simulink model "MVDR_example_hdl_4x4_systolic"  (R2020a)
settings: Solver=FixedStepDiscrete  StartTime=0.0  StopTime=stoptime  RelTol=1e-3
InitFcn:
  | model_init
values from neighbouring files (symbols this model uses):
  BackSubstitutePrototype = fi(0, matrixdivbacksub_dt)    [model_init.m]
  matrixDivDelay = NumberOfCORDICIterations*10 + 86    [model_init.m]
  movavg_bitshift = nextpow2(sqrt(windowSize))    [model_init.m]
  mvdrPipelineDelay = covMatDelay+movAvgDelay+matrixDivDelay+normResponseDelay    [model_init.m]
  numArrayElements = 4    [model_init.m]
  NumberOfCORDICIterations = matrixdivin_dt.WordLength - 1    [model_init.m]
  srcAngles = [20 60]    [model_init.m]
  sv = step(steeringVector,fc,[scanAngle; 0])    [model_init.m]
  Ts = 1/fs    (= 7.8125e-09)    [model_init.m]
  windowSize = 1024    [model_init.m]
libraries: hdlsllib x249, simulink x44, commfilt2 x4, commrfcorlib x3, commsync2 x3, commrflib2 x2, commrandsrc3 x2, phasedtxrxlib x2, commdigbbndcpm2 x1, dspsolvers x1, embreciprocals x1, commdigbbndpm3 x1
(part 7 of 11)

== system MVDR_example_hdl_4x4_systolic/MVDR HDL/Compute Weight Vector/Matrix Left Divide/CORDIC/4x4 Complex CORDIC Matrix Left Divide/Q'B, R 4x4 Complex CORDIC Systolic Array/Leading Complex Row Rotation/Rotate first element to real/Inverse CORDIC Gain2 ==
  In1 : Inport
  Inverse CORDIC Gain : Gain  Gain=1/prod(sqrt(1+2.^(-2*(0:double(NumberOfCORDICIterations)-1))))  OutDataTypeStr=Inherit: Same as input
  Out1 : Outport  VectorParamsAs1DForOutWhenUnconnected=off
  wires:
  Inverse CORDIC Gain/1 -> Out1/1
  In1/1 -> Inverse CORDIC Gain/1

== system MVDR_example_hdl_4x4_systolic/MVDR HDL/Compute Weight Vector/Matrix Left Divide/CORDIC/4x4 Complex CORDIC Matrix Left Divide/Q'B, R 4x4 Complex CORDIC Systolic Array/Leading Complex Row Rotation/Rotate first element to real/Inverse CORDIC Gain3 ==
  In1 : Inport
  Inverse CORDIC Gain : Gain  Gain=1/prod(sqrt(1+2.^(-2*(0:double(NumberOfCORDICIterations)-1))))  OutDataTypeStr=Inherit: Same as input
  Out1 : Outport  VectorParamsAs1DForOutWhenUnconnected=off
  wires:
  Inverse CORDIC Gain/1 -> Out1/1
  In1/1 -> Inverse CORDIC Gain/1

== system MVDR_example_hdl_4x4_systolic/MVDR HDL/Compute Weight Vector/Matrix Left Divide/CORDIC/4x4 Complex CORDIC Matrix Left Divide/Q'B, R 4x4 Complex CORDIC Systolic Array/Leading Complex Row Rotation/Rotate first element to real/Inverse CORDIC Gain4 ==
  In1 : Inport
  Inverse CORDIC Gain : Gain  Gain=1/prod(sqrt(1+2.^(-2*(0:double(NumberOfCORDICIterations)-1))))  OutDataTypeStr=Inherit: Same as input
  Out1 : Outport  VectorParamsAs1DForOutWhenUnconnected=off
  wires:
  Inverse CORDIC Gain/1 -> Out1/1
  In1/1 -> Inverse CORDIC Gain/1

== system MVDR_example_hdl_4x4_systolic/MVDR HDL/Compute Weight Vector/Matrix Left Divide/CORDIC/4x4 Complex CORDIC Matrix Left Divide/Q'B, R 4x4 Complex CORDIC Systolic Array/Leading Complex Row Rotation/Rotate first element to real/Q'B, R Row Rotations - Real ==
  x : Inport
  y : Inport  Port=2
  u : Inport  Port=3
  v : Inport  Port=4
  validIn : Inport  Port=5
  CORDIC Counter : Subsystem  mask{NumberOfCORDICIterations=NumberOfCORDICIterations}
      mask prompts: NumberOfCORDICIterations "Number of CORDIC Iterations"
  Delay{1..12} (12 alike) : Delay  DelayLength=1
  Delay13 : Delay  DelayLength=1  InitialCondition=true
  MATLAB Function : MATLAB Function  TreatAsAtomicUnit=on
  Same Datatype : Subsystem  TreatAsAtomicUnit=on
  Same Datatype1 : Subsystem  TreatAsAtomicUnit=on
  Same Datatype2 : Subsystem  TreatAsAtomicUnit=on
  Same Datatype3 : Subsystem  TreatAsAtomicUnit=on
  State Control : StateControl  StateControl=Synchronous
  Switch{,1..3} (4 alike) : Switch  Criteria=u2 ~= 0
  x_out : Outport  VectorParamsAs1DForOutWhenUnconnected=off
  y_out : Outport  Port=2  VectorParamsAs1DForOutWhenUnconnected=off
  u_out : Outport  Port=3  VectorParamsAs1DForOutWhenUnconnected=off
  v_out : Outport  Port=4  VectorParamsAs1DForOutWhenUnconnected=off
  validOut : Outport  Port=5  VectorParamsAs1DForOutWhenUnconnected=off
  ready : Outport  Port=6  VectorParamsAs1DForOutWhenUnconnected=off
  wires:
  Delay13/1 -> ready/1
  Delay12/1 -> Delay3/1
  Delay10/1 -> MATLAB Function/5(iteration)
  Delay9/1 -> Switch/2, Switch1/2, Switch2/2, Switch3/2
  Delay8/1 -> Same Datatype2/2(Reference), Switch3/3
  Delay6/1 -> Same Datatype3/2(Reference), Switch2/3
  Delay5/1 -> Same Datatype1/2(Reference), Switch1/3
  Delay4/1 -> Same Datatype/2(Reference), Switch/3
  Delay1/1 -> Same Datatype/1(Data), x_out/1
  Delay2/1 -> Same Datatype1/1(Data), y_out/1
  Delay11/1 -> Same Datatype2/1(Data), v_out/1
  MATLAB Function/1(x_out) -> Delay1/1
  MATLAB Function/2(y_out) -> Delay2/1
  MATLAB Function/3(u_out) -> Delay7/1
  MATLAB Function/4(v_out) -> Delay11/1
  Delay7/1 -> Same Datatype3/1(Data), u_out/1
  Delay3/1 -> validOut/1
  validIn/1 -> CORDIC Counter/1(validIn)
  CORDIC Counter/2(count) -> Delay10/1
  CORDIC Counter/3(last) -> Delay12/1
  CORDIC Counter/4(ready) -> Delay13/1
  Switch/1 -> MATLAB Function/1(x)
  Switch1/1 -> MATLAB Function/2(y)
  Switch2/1 -> MATLAB Function/3(u)
  Switch3/1 -> MATLAB Function/4(v)
  CORDIC Counter/1(count_is_positive) -> Delay9/1
  x/1 -> Delay4/1
  y/1 -> Delay5/1
  u/1 -> Delay6/1
  v/1 -> Delay8/1
  Same Datatype/1(DataOut) -> Switch/1
  Same Datatype1/1(DataOut) -> Switch1/1
  Same Datatype3/1(DataOut) -> Switch2/1
  Same Datatype2/1(DataOut) -> Switch3/1

== system MVDR_example_hdl_4x4_systolic/MVDR HDL/Compute Weight Vector/Matrix Left Divide/CORDIC/4x4 Complex CORDIC Matrix Left Divide/Q'B, R 4x4 Complex CORDIC Systolic Array/Leading Complex Row Rotation/Rotate first element to real/ValidIn to Ready Logic with Delay ==
  readyIn : Inport
  validIn * z^-1 : Inport  Port=2
  validIn : Inport  Port=3
  AND : Logic  IconShape=distinctive  AllPortsSameDT=off  OutDataTypeStr=boolean
  AND1 : Logic  IconShape=distinctive  AllPortsSameDT=off  OutDataTypeStr=boolean
  NOT : Logic  Operator=NOT  IconShape=distinctive  AllPortsSameDT=off  OutDataTypeStr=boolean
  NOT1 : Logic  Operator=NOT  IconShape=distinctive  AllPortsSameDT=off  OutDataTypeStr=boolean
  readyOut : Outport  VectorParamsAs1DForOutWhenUnconnected=off
  wires:
  validIn * z^-1/1 -> NOT/1
  validIn/1 -> NOT1/1
  readyIn/1 -> AND/1
  AND1/1 -> readyOut/1
  NOT1/1 -> AND1/2
  NOT/1 -> AND/2
  AND/1 -> AND1/1

== system MVDR_example_hdl_4x4_systolic/MVDR HDL/Compute Weight Vector/Matrix Left Divide/CORDIC/4x4 Complex CORDIC Matrix Left Divide/Q'B, R 4x4 Complex CORDIC Systolic Array/Leading Complex Row Rotation/Rotate first element to real - 1/Inverse CORDIC Gain1 ==
  In1 : Inport
  Inverse CORDIC Gain : Gain  Gain=1/prod(sqrt(1+2.^(-2*(0:double(NumberOfCORDICIterations)-1))))  OutDataTypeStr=Inherit: Same as input
  Out1 : Outport  VectorParamsAs1DForOutWhenUnconnected=off
  wires:
  Inverse CORDIC Gain/1 -> Out1/1
  In1/1 -> Inverse CORDIC Gain/1

== system MVDR_example_hdl_4x4_systolic/MVDR HDL/Compute Weight Vector/Matrix Left Divide/CORDIC/4x4 Complex CORDIC Matrix Left Divide/Q'B, R 4x4 Complex CORDIC Systolic Array/Leading Complex Row Rotation/Rotate first element to real - 1/Inverse CORDIC Gain2 ==
  In1 : Inport
  Inverse CORDIC Gain : Gain  Gain=1/prod(sqrt(1+2.^(-2*(0:double(NumberOfCORDICIterations)-1))))  OutDataTypeStr=Inherit: Same as input
  Out1 : Outport  VectorParamsAs1DForOutWhenUnconnected=off
  wires:
  Inverse CORDIC Gain/1 -> Out1/1
  In1/1 -> Inverse CORDIC Gain/1

== system MVDR_example_hdl_4x4_systolic/MVDR HDL/Compute Weight Vector/Matrix Left Divide/CORDIC/4x4 Complex CORDIC Matrix Left Divide/Q'B, R 4x4 Complex CORDIC Systolic Array/Leading Complex Row Rotation/Rotate first element to real - 1/Inverse CORDIC Gain3 ==
  In1 : Inport
  Inverse CORDIC Gain : Gain  Gain=1/prod(sqrt(1+2.^(-2*(0:double(NumberOfCORDICIterations)-1))))  OutDataTypeStr=Inherit: Same as input
  Out1 : Outport  VectorParamsAs1DForOutWhenUnconnected=off
  wires:
  Inverse CORDIC Gain/1 -> Out1/1
  In1/1 -> Inverse CORDIC Gain/1

== system MVDR_example_hdl_4x4_systolic/MVDR HDL/Compute Weight Vector/Matrix Left Divide/CORDIC/4x4 Complex CORDIC Matrix Left Divide/Q'B, R 4x4 Complex CORDIC Systolic Array/Leading Complex Row Rotation/Rotate first element to real - 1/Inverse CORDIC Gain4 ==
  In1 : Inport
  Inverse CORDIC Gain : Gain  Gain=1/prod(sqrt(1+2.^(-2*(0:double(NumberOfCORDICIterations)-1))))  OutDataTypeStr=Inherit: Same as input
  Out1 : Outport  VectorParamsAs1DForOutWhenUnconnected=off
  wires:
  Inverse CORDIC Gain/1 -> Out1/1
  In1/1 -> Inverse CORDIC Gain/1

== system MVDR_example_hdl_4x4_systolic/MVDR HDL/Compute Weight Vector/Matrix Left Divide/CORDIC/4x4 Complex CORDIC Matrix Left Divide/Q'B, R 4x4 Complex CORDIC Systolic Array/Leading Complex Row Rotation/Rotate first element to real - 1/Q'B, R Row Rotations - Real ==
  x : Inport
  y : Inport  Port=2
  u : Inport  Port=3
  v : Inport  Port=4
  validIn : Inport  Port=5
  CORDIC Counter : Subsystem  mask{NumberOfCORDICIterations=NumberOfCORDICIterations}
      mask prompts: NumberOfCORDICIterations "Number of CORDIC Iterations"
  Delay{1..12} (12 alike) : Delay  DelayLength=1
  Delay13 : Delay  DelayLength=1  InitialCondition=true
  MATLAB Function : MATLAB Function  TreatAsAtomicUnit=on
  Same Datatype : Subsystem  TreatAsAtomicUnit=on
  Same Datatype1 : Subsystem  TreatAsAtomicUnit=on
  Same Datatype2 : Subsystem  TreatAsAtomicUnit=on
  Same Datatype3 : Subsystem  TreatAsAtomicUnit=on
  State Control : StateControl  StateControl=Synchronous
  Switch{,1..3} (4 alike) : Switch  Criteria=u2 ~= 0
  x_out : Outport  VectorParamsAs1DForOutWhenUnconnected=off
  y_out : Outport  Port=2  VectorParamsAs1DForOutWhenUnconnected=off
  u_out : Outport  Port=3  VectorParamsAs1DForOutWhenUnconnected=off
  v_out : Outport  Port=4  VectorParamsAs1DForOutWhenUnconnected=off
  validOut : Outport  Port=5  VectorParamsAs1DForOutWhenUnconnected=off
  ready : Outport  Port=6  VectorParamsAs1DForOutWhenUnconnected=off
  wires:
  Delay13/1 -> ready/1
  Delay12/1 -> Delay3/1
  Delay10/1 -> MATLAB Function/5(iteration)
  Delay9/1 -> Switch/2, Switch1/2, Switch2/2, Switch3/2
  Delay8/1 -> Same Datatype2/2(Reference), Switch3/3
  Delay6/1 -> Same Datatype3/2(Reference), Switch2/3
  Delay5/1 -> Same Datatype1/2(Reference), Switch1/3
  Delay4/1 -> Same Datatype/2(Reference), Switch/3
  Delay1/1 -> Same Datatype/1(Data), x_out/1
  Delay2/1 -> Same Datatype1/1(Data), y_out/1
  Delay11/1 -> Same Datatype2/1(Data), v_out/1
  MATLAB Function/1(x_out) -> Delay1/1
  MATLAB Function/2(y_out) -> Delay2/1
  MATLAB Function/3(u_out) -> Delay7/1
  MATLAB Function/4(v_out) -> Delay11/1
  Delay7/1 -> Same Datatype3/1(Data), u_out/1
  Delay3/1 -> validOut/1
  validIn/1 -> CORDIC Counter/1(validIn)
  CORDIC Counter/2(count) -> Delay10/1
  CORDIC Counter/3(last) -> Delay12/1
  CORDIC Counter/4(ready) -> Delay13/1
  Switch/1 -> MATLAB Function/1(x)
  Switch1/1 -> MATLAB Function/2(y)
  Switch2/1 -> MATLAB Function/3(u)
  Switch3/1 -> MATLAB Function/4(v)
  CORDIC Counter/1(count_is_positive) -> Delay9/1
  x/1 -> Delay4/1
  y/1 -> Delay5/1
  u/1 -> Delay6/1
  v/1 -> Delay8/1
  Same Datatype/1(DataOut) -> Switch/1
  Same Datatype1/1(DataOut) -> Switch1/1
  Same Datatype3/1(DataOut) -> Switch2/1
  Same Datatype2/1(DataOut) -> Switch3/1

== system MVDR_example_hdl_4x4_systolic/MVDR HDL/Compute Weight Vector/Matrix Left Divide/CORDIC/4x4 Complex CORDIC Matrix Left Divide/Q'B, R 4x4 Complex CORDIC Systolic Array/Leading Complex Row Rotation/Rotate first element to real - 1/ValidIn to Ready Logic with Delay ==
  readyIn : Inport
  validIn * z^-1 : Inport  Port=2
  validIn : Inport  Port=3
  AND : Logic  IconShape=distinctive  AllPortsSameDT=off  OutDataTypeStr=boolean
  AND1 : Logic  IconShape=distinctive  AllPortsSameDT=off  OutDataTypeStr=boolean
  NOT : Logic  Operator=NOT  IconShape=distinctive  AllPortsSameDT=off  OutDataTypeStr=boolean
  NOT1 : Logic  Operator=NOT  IconShape=distinctive  AllPortsSameDT=off  OutDataTypeStr=boolean
  readyOut : Outport  VectorParamsAs1DForOutWhenUnconnected=off
  wires:
  validIn * z^-1/1 -> NOT/1
  validIn/1 -> NOT1/1
  readyIn/1 -> AND/1
  AND1/1 -> readyOut/1
  NOT1/1 -> AND1/2
  NOT/1 -> AND/2
  AND/1 -> AND1/1

== system MVDR_example_hdl_4x4_systolic/MVDR HDL/Compute Weight Vector/Matrix Left Divide/CORDIC/4x4 Complex CORDIC Matrix Left Divide/Q'B, R 4x4 Complex CORDIC Systolic Array/Leading Complex Row Rotation - 2/Q'B, R Row Rotations - Complex/CORDIC Counter ==
  validIn : Inport
  Compare To Constant : simulink/Logic and Bit Operations/Compare To Constant  relop===  const=NumberOfCORDICIterations-1  OutDataTypeStr=boolean
  Compare To Zero : simulink/Logic and Bit Operations/Compare To Zero  relop=>  OutDataTypeStr=boolean
  HDL Counter1 : hdlsllib/Sources/HDL Counter  CountType=Count limited  CountInit=0  CountStep=1  CountMax=NumberOfCORDICIterations-1  CountFromType=Initial value  CountFrom=0  CountResetPort=off  CountLoadPort=off  CountEnbPort=on  CountDirPort=off  CountDataType=Unsigned  CountWordLen=nextpow2(NumberOfCORDICIterations)  CountFracLen=0  CountSampTime=1
  OR : Logic  Operator=OR  IconShape=distinctive  AllPortsSameDT=off  OutDataTypeStr=boolean
  SR_latch : Subsystem
  State Control : StateControl  StateControl=Synchronous
  ValidIn to Ready Logic : Subsystem
  count_is_positive : Outport  VectorParamsAs1DForOutWhenUnconnected=off
  count : Outport  Port=2  VectorParamsAs1DForOutWhenUnconnected=off
  last : Outport  Port=3  VectorParamsAs1DForOutWhenUnconnected=off
  ready : Outport  Port=4  VectorParamsAs1DForOutWhenUnconnected=off
  wires:
  HDL Counter1/1 -> Compare To Zero/1, count/1, Compare To Constant/1  "count"
  OR/1 -> HDL Counter1/1
  Compare To Zero/1 -> count_is_positive/1, OR/1
  Compare To Constant/1 -> SR_latch/1(S), last/1
  validIn/1 -> ValidIn to Ready Logic/2(validIn), SR_latch/2(R), OR/2
  SR_latch/1(Q) -> ValidIn to Ready Logic/1(readyIn)  "ready"
  ValidIn to Ready Logic/1(readyOut) -> ready/1

== system MVDR_example_hdl_4x4_systolic/MVDR HDL/Compute Weight Vector/Matrix Left Divide/CORDIC/4x4 Complex CORDIC Matrix Left Divide/Q'B, R 4x4 Complex CORDIC Systolic Array/Leading Complex Row Rotation - 2/Q'B, R Row Rotations - Complex/Same Datatype ==
  Data : Inport
  Reference : Inport  Port=2
  Data Type Duplicate : DataTypeDuplicate
  DataOut : Outport  VectorParamsAs1DForOutWhenUnconnected=off
  wires:
  Data/1 -> Data Type Duplicate/1, DataOut/1
  Reference/1 -> Data Type Duplicate/2

== system MVDR_example_hdl_4x4_systolic/MVDR HDL/Compute Weight Vector/Matrix Left Divide/CORDIC/4x4 Complex CORDIC Matrix Left Divide/Q'B, R 4x4 Complex CORDIC Systolic Array/Leading Complex Row Rotation - 2/Q'B, R Row Rotations - Complex/Same Datatype1 ==
  Data : Inport
  Reference : Inport  Port=2
  Data Type Duplicate : DataTypeDuplicate
  DataOut : Outport  VectorParamsAs1DForOutWhenUnconnected=off
  wires:
  Data/1 -> Data Type Duplicate/1, DataOut/1
  Reference/1 -> Data Type Duplicate/2

== system MVDR_example_hdl_4x4_systolic/MVDR HDL/Compute Weight Vector/Matrix Left Divide/CORDIC/4x4 Complex CORDIC Matrix Left Divide/Q'B, R 4x4 Complex CORDIC Systolic Array/Leading Complex Row Rotation - 2/Q'B, R Row Rotations - Complex/Same Datatype2 ==
  Data : Inport
  Reference : Inport  Port=2
  Data Type Duplicate : DataTypeDuplicate
  DataOut : Outport  VectorParamsAs1DForOutWhenUnconnected=off
  wires:
  Data/1 -> Data Type Duplicate/1, DataOut/1
  Reference/1 -> Data Type Duplicate/2

== system MVDR_example_hdl_4x4_systolic/MVDR HDL/Compute Weight Vector/Matrix Left Divide/CORDIC/4x4 Complex CORDIC Matrix Left Divide/Q'B, R 4x4 Complex CORDIC Systolic Array/Leading Complex Row Rotation - 2/Q'B, R Row Rotations - Complex/Same Datatype3 ==
  Data : Inport
  Reference : Inport  Port=2
  Data Type Duplicate : DataTypeDuplicate
  DataOut : Outport  VectorParamsAs1DForOutWhenUnconnected=off
  wires:
  Data/1 -> Data Type Duplicate/1, DataOut/1
  Reference/1 -> Data Type Duplicate/2

== system MVDR_example_hdl_4x4_systolic/MVDR HDL/Compute Weight Vector/Matrix Left Divide/CORDIC/4x4 Complex CORDIC Matrix Left Divide/Q'B, R 4x4 Complex CORDIC Systolic Array/Leading Complex Row Rotation - 2/Rotate first element to real/Inverse CORDIC Gain1 ==
  In1 : Inport
  Inverse CORDIC Gain : Gain  Gain=1/prod(sqrt(1+2.^(-2*(0:double(NumberOfCORDICIterations)-1))))  OutDataTypeStr=Inherit: Same as input
  Out1 : Outport  VectorParamsAs1DForOutWhenUnconnected=off
  wires:
  Inverse CORDIC Gain/1 -> Out1/1
  In1/1 -> Inverse CORDIC Gain/1

== system MVDR_example_hdl_4x4_systolic/MVDR HDL/Compute Weight Vector/Matrix Left Divide/CORDIC/4x4 Complex CORDIC Matrix Left Divide/Q'B, R 4x4 Complex CORDIC Systolic Array/Leading Complex Row Rotation - 2/Rotate first element to real/Inverse CORDIC Gain2 ==
  In1 : Inport
  Inverse CORDIC Gain : Gain  Gain=1/prod(sqrt(1+2.^(-2*(0:double(NumberOfCORDICIterations)-1))))  OutDataTypeStr=Inherit: Same as input
  Out1 : Outport  VectorParamsAs1DForOutWhenUnconnected=off
  wires:
  Inverse CORDIC Gain/1 -> Out1/1
  In1/1 -> Inverse CORDIC Gain/1

== system MVDR_example_hdl_4x4_systolic/MVDR HDL/Compute Weight Vector/Matrix Left Divide/CORDIC/4x4 Complex CORDIC Matrix Left Divide/Q'B, R 4x4 Complex CORDIC Systolic Array/Leading Complex Row Rotation - 2/Rotate first element to real/Inverse CORDIC Gain3 ==
  In1 : Inport
  Inverse CORDIC Gain : Gain  Gain=1/prod(sqrt(1+2.^(-2*(0:double(NumberOfCORDICIterations)-1))))  OutDataTypeStr=Inherit: Same as input
  Out1 : Outport  VectorParamsAs1DForOutWhenUnconnected=off
  wires:
  Inverse CORDIC Gain/1 -> Out1/1
  In1/1 -> Inverse CORDIC Gain/1

== system MVDR_example_hdl_4x4_systolic/MVDR HDL/Compute Weight Vector/Matrix Left Divide/CORDIC/4x4 Complex CORDIC Matrix Left Divide/Q'B, R 4x4 Complex CORDIC Systolic Array/Leading Complex Row Rotation - 2/Rotate first element to real/Inverse CORDIC Gain4 ==
  In1 : Inport
  Inverse CORDIC Gain : Gain  Gain=1/prod(sqrt(1+2.^(-2*(0:double(NumberOfCORDICIterations)-1))))  OutDataTypeStr=Inherit: Same as input
  Out1 : Outport  VectorParamsAs1DForOutWhenUnconnected=off
  wires:
  Inverse CORDIC Gain/1 -> Out1/1
  In1/1 -> Inverse CORDIC Gain/1

== system MVDR_example_hdl_4x4_systolic/MVDR HDL/Compute Weight Vector/Matrix Left Divide/CORDIC/4x4 Complex CORDIC Matrix Left Divide/Q'B, R 4x4 Complex CORDIC Systolic Array/Leading Complex Row Rotation - 2/Rotate first element to real/Q'B, R Row Rotations - Real ==
  x : Inport
  y : Inport  Port=2
  u : Inport  Port=3
  v : Inport  Port=4
  validIn : Inport  Port=5
  CORDIC Counter : Subsystem  mask{NumberOfCORDICIterations=NumberOfCORDICIterations}
      mask prompts: NumberOfCORDICIterations "Number of CORDIC Iterations"
  Delay{1..12} (12 alike) : Delay  DelayLength=1
  Delay13 : Delay  DelayLength=1  InitialCondition=true
  MATLAB Function : MATLAB Function  TreatAsAtomicUnit=on
  Same Datatype : Subsystem  TreatAsAtomicUnit=on
  Same Datatype1 : Subsystem  TreatAsAtomicUnit=on
  Same Datatype2 : Subsystem  TreatAsAtomicUnit=on
  Same Datatype3 : Subsystem  TreatAsAtomicUnit=on
  State Control : StateControl  StateControl=Synchronous
  Switch{,1..3} (4 alike) : Switch  Criteria=u2 ~= 0
  x_out : Outport  VectorParamsAs1DForOutWhenUnconnected=off
  y_out : Outport  Port=2  VectorParamsAs1DForOutWhenUnconnected=off
  u_out : Outport  Port=3  VectorParamsAs1DForOutWhenUnconnected=off
  v_out : Outport  Port=4  VectorParamsAs1DForOutWhenUnconnected=off
  validOut : Outport  Port=5  VectorParamsAs1DForOutWhenUnconnected=off
  ready : Outport  Port=6  VectorParamsAs1DForOutWhenUnconnected=off
  wires:
  Delay13/1 -> ready/1
  Delay12/1 -> Delay3/1
  Delay10/1 -> MATLAB Function/5(iteration)
  Delay9/1 -> Switch/2, Switch1/2, Switch2/2, Switch3/2
  Delay8/1 -> Same Datatype2/2(Reference), Switch3/3
  Delay6/1 -> Same Datatype3/2(Reference), Switch2/3
  Delay5/1 -> Same Datatype1/2(Reference), Switch1/3
  Delay4/1 -> Same Datatype/2(Reference), Switch/3
  Delay1/1 -> Same Datatype/1(Data), x_out/1
  Delay2/1 -> Same Datatype1/1(Data), y_out/1
  Delay11/1 -> Same Datatype2/1(Data), v_out/1
  MATLAB Function/1(x_out) -> Delay1/1
  MATLAB Function/2(y_out) -> Delay2/1
  MATLAB Function/3(u_out) -> Delay7/1
  MATLAB Function/4(v_out) -> Delay11/1
  Delay7/1 -> Same Datatype3/1(Data), u_out/1
  Delay3/1 -> validOut/1
  validIn/1 -> CORDIC Counter/1(validIn)
  CORDIC Counter/2(count) -> Delay10/1
  CORDIC Counter/3(last) -> Delay12/1
  CORDIC Counter/4(ready) -> Delay13/1
  Switch/1 -> MATLAB Function/1(x)
  Switch1/1 -> MATLAB Function/2(y)
  Switch2/1 -> MATLAB Function/3(u)
  Switch3/1 -> MATLAB Function/4(v)
  CORDIC Counter/1(count_is_positive) -> Delay9/1
  x/1 -> Delay4/1
  y/1 -> Delay5/1
  u/1 -> Delay6/1
  v/1 -> Delay8/1
  Same Datatype/1(DataOut) -> Switch/1
  Same Datatype1/1(DataOut) -> Switch1/1
  Same Datatype3/1(DataOut) -> Switch2/1
  Same Datatype2/1(DataOut) -> Switch3/1

== system MVDR_example_hdl_4x4_systolic/MVDR HDL/Compute Weight Vector/Matrix Left Divide/CORDIC/4x4 Complex CORDIC Matrix Left Divide/Q'B, R 4x4 Complex CORDIC Systolic Array/Leading Complex Row Rotation - 2/Rotate first element to real/ValidIn to Ready Logic with Delay ==
  readyIn : Inport
  validIn * z^-1 : Inport  Port=2
  validIn : Inport  Port=3
  AND : Logic  IconShape=distinctive  AllPortsSameDT=off  OutDataTypeStr=boolean
  AND1 : Logic  IconShape=distinctive  AllPortsSameDT=off  OutDataTypeStr=boolean
  NOT : Logic  Operator=NOT  IconShape=distinctive  AllPortsSameDT=off  OutDataTypeStr=boolean
  NOT1 : Logic  Operator=NOT  IconShape=distinctive  AllPortsSameDT=off  OutDataTypeStr=boolean
  readyOut : Outport  VectorParamsAs1DForOutWhenUnconnected=off
  wires:
  validIn * z^-1/1 -> NOT/1
  validIn/1 -> NOT1/1
  readyIn/1 -> AND/1
  AND1/1 -> readyOut/1
  NOT1/1 -> AND1/2
  NOT/1 -> AND/2
  AND/1 -> AND1/1

== system MVDR_example_hdl_4x4_systolic/MVDR HDL/Compute Weight Vector/Matrix Left Divide/CORDIC/4x4 Complex CORDIC Matrix Left Divide/Q'B, R 4x4 Complex CORDIC Systolic Array/Leading Complex Row Rotation - 2/Rotate first element to real - 1/Inverse CORDIC Gain1 ==
  In1 : Inport
  Inverse CORDIC Gain : Gain  Gain=1/prod(sqrt(1+2.^(-2*(0:double(NumberOfCORDICIterations)-1))))  OutDataTypeStr=Inherit: Same as input
  Out1 : Outport  VectorParamsAs1DForOutWhenUnconnected=off
  wires:
  Inverse CORDIC Gain/1 -> Out1/1
  In1/1 -> Inverse CORDIC Gain/1

== system MVDR_example_hdl_4x4_systolic/MVDR HDL/Compute Weight Vector/Matrix Left Divide/CORDIC/4x4 Complex CORDIC Matrix Left Divide/Q'B, R 4x4 Complex CORDIC Systolic Array/Leading Complex Row Rotation - 2/Rotate first element to real - 1/Inverse CORDIC Gain2 ==
  In1 : Inport
  Inverse CORDIC Gain : Gain  Gain=1/prod(sqrt(1+2.^(-2*(0:double(NumberOfCORDICIterations)-1))))  OutDataTypeStr=Inherit: Same as input
  Out1 : Outport  VectorParamsAs1DForOutWhenUnconnected=off
  wires:
  Inverse CORDIC Gain/1 -> Out1/1
  In1/1 -> Inverse CORDIC Gain/1

== system MVDR_example_hdl_4x4_systolic/MVDR HDL/Compute Weight Vector/Matrix Left Divide/CORDIC/4x4 Complex CORDIC Matrix Left Divide/Q'B, R 4x4 Complex CORDIC Systolic Array/Leading Complex Row Rotation - 2/Rotate first element to real - 1/Inverse CORDIC Gain3 ==
  In1 : Inport
  Inverse CORDIC Gain : Gain  Gain=1/prod(sqrt(1+2.^(-2*(0:double(NumberOfCORDICIterations)-1))))  OutDataTypeStr=Inherit: Same as input
  Out1 : Outport  VectorParamsAs1DForOutWhenUnconnected=off
  wires:
  Inverse CORDIC Gain/1 -> Out1/1
  In1/1 -> Inverse CORDIC Gain/1

== system MVDR_example_hdl_4x4_systolic/MVDR HDL/Compute Weight Vector/Matrix Left Divide/CORDIC/4x4 Complex CORDIC Matrix Left Divide/Q'B, R 4x4 Complex CORDIC Systolic Array/Leading Complex Row Rotation - 2/Rotate first element to real - 1/Inverse CORDIC Gain4 ==
  In1 : Inport
  Inverse CORDIC Gain : Gain  Gain=1/prod(sqrt(1+2.^(-2*(0:double(NumberOfCORDICIterations)-1))))  OutDataTypeStr=Inherit: Same as input
  Out1 : Outport  VectorParamsAs1DForOutWhenUnconnected=off
  wires:
  Inverse CORDIC Gain/1 -> Out1/1
  In1/1 -> Inverse CORDIC Gain/1

== system MVDR_example_hdl_4x4_systolic/MVDR HDL/Compute Weight Vector/Matrix Left Divide/CORDIC/4x4 Complex CORDIC Matrix Left Divide/Q'B, R 4x4 Complex CORDIC Systolic Array/Leading Complex Row Rotation - 2/Rotate first element to real - 1/Q'B, R Row Rotations - Real ==
  x : Inport
  y : Inport  Port=2
  u : Inport  Port=3
  v : Inport  Port=4
  validIn : Inport  Port=5
  CORDIC Counter : Subsystem  mask{NumberOfCORDICIterations=NumberOfCORDICIterations}
      mask prompts: NumberOfCORDICIterations "Number of CORDIC Iterations"
  Delay{1..12} (12 alike) : Delay  DelayLength=1
  Delay13 : Delay  DelayLength=1  InitialCondition=true
  MATLAB Function : MATLAB Function  TreatAsAtomicUnit=on
  Same Datatype : Subsystem  TreatAsAtomicUnit=on
  Same Datatype1 : Subsystem  TreatAsAtomicUnit=on
  Same Datatype2 : Subsystem  TreatAsAtomicUnit=on
  Same Datatype3 : Subsystem  TreatAsAtomicUnit=on
  State Control : StateControl  StateControl=Synchronous
  Switch{,1..3} (4 alike) : Switch  Criteria=u2 ~= 0
  x_out : Outport  VectorParamsAs1DForOutWhenUnconnected=off
  y_out : Outport  Port=2  VectorParamsAs1DForOutWhenUnconnected=off
  u_out : Outport  Port=3  VectorParamsAs1DForOutWhenUnconnected=off
  v_out : Outport  Port=4  VectorParamsAs1DForOutWhenUnconnected=off
  validOut : Outport  Port=5  VectorParamsAs1DForOutWhenUnconnected=off
  ready : Outport  Port=6  VectorParamsAs1DForOutWhenUnconnected=off
  wires:
  Same Datatype2/1(DataOut) -> Switch3/1
  Same Datatype3/1(DataOut) -> Switch2/1
  Same Datatype1/1(DataOut) -> Switch1/1
  Same Datatype/1(DataOut) -> Switch/1
  v/1 -> Delay8/1
  u/1 -> Delay6/1
  y/1 -> Delay5/1
  x/1 -> Delay4/1
  CORDIC Counter/1(count_is_positive) -> Delay9/1
  Switch3/1 -> MATLAB Function/4(v)
  Switch2/1 -> MATLAB Function/3(u)
  Switch1/1 -> MATLAB Function/2(y)
  Switch/1 -> MATLAB Function/1(x)
  CORDIC Counter/4(ready) -> Delay13/1
  CORDIC Counter/3(last) -> Delay12/1
  CORDIC Counter/2(count) -> Delay10/1
  validIn/1 -> CORDIC Counter/1(validIn)
  Delay3/1 -> validOut/1
  Delay7/1 -> u_out/1, Same Datatype3/1(Data)
  MATLAB Function/4(v_out) -> Delay11/1
  MATLAB Function/3(u_out) -> Delay7/1
  MATLAB Function/2(y_out) -> Delay2/1
  MATLAB Function/1(x_out) -> Delay1/1
  Delay11/1 -> v_out/1, Same Datatype2/1(Data)
  Delay2/1 -> y_out/1, Same Datatype1/1(Data)
  Delay1/1 -> x_out/1, Same Datatype/1(Data)
  Delay4/1 -> Switch/3, Same Datatype/2(Reference)
  Delay5/1 -> Switch1/3, Same Datatype1/2(Reference)
  Delay6/1 -> Switch2/3, Same Datatype3/2(Reference)
  Delay8/1 -> Switch3/3, Same Datatype2/2(Reference)
  Delay9/1 -> Switch3/2, Switch2/2, Switch1/2, Switch/2
  Delay10/1 -> MATLAB Function/5(iteration)
  Delay12/1 -> Delay3/1
  Delay13/1 -> ready/1

== system MVDR_example_hdl_4x4_systolic/MVDR HDL/Compute Weight Vector/Matrix Left Divide/CORDIC/4x4 Complex CORDIC Matrix Left Divide/Q'B, R 4x4 Complex CORDIC Systolic Array/Leading Complex Row Rotation - 2/Rotate first element to real - 1/ValidIn to Ready Logic with Delay ==
  readyIn : Inport
  validIn * z^-1 : Inport  Port=2
  validIn : Inport  Port=3
  AND : Logic  IconShape=distinctive  AllPortsSameDT=off  OutDataTypeStr=boolean
  AND1 : Logic  IconShape=distinctive  AllPortsSameDT=off  OutDataTypeStr=boolean
  NOT : Logic  Operator=NOT  IconShape=distinctive  AllPortsSameDT=off  OutDataTypeStr=boolean
  NOT1 : Logic  Operator=NOT  IconShape=distinctive  AllPortsSameDT=off  OutDataTypeStr=boolean
  readyOut : Outport  VectorParamsAs1DForOutWhenUnconnected=off
  wires:
  validIn * z^-1/1 -> NOT/1
  validIn/1 -> NOT1/1
  readyIn/1 -> AND/1
  AND1/1 -> readyOut/1
  NOT1/1 -> AND1/2
  NOT/1 -> AND/2
  AND/1 -> AND1/1

== system MVDR_example_hdl_4x4_systolic/MVDR HDL/Compute Weight Vector/Matrix Left Divide/CORDIC/4x4 Complex CORDIC Matrix Left Divide/Q'B, R 4x4 Complex CORDIC Systolic Array/Leading Complex Row Rotation - 3/Q'B, R Row Rotations - Complex/CORDIC Counter ==
  validIn : Inport
  Compare To Constant : simulink/Logic and Bit Operations/Compare To Constant  relop===  const=NumberOfCORDICIterations-1  OutDataTypeStr=boolean
  Compare To Zero : simulink/Logic and Bit Operations/Compare To Zero  relop=>  OutDataTypeStr=boolean
  HDL Counter1 : hdlsllib/Sources/HDL Counter  CountType=Count limited  CountInit=0  CountStep=1  CountMax=NumberOfCORDICIterations-1  CountFromType=Initial value  CountFrom=0  CountResetPort=off  CountLoadPort=off  CountEnbPort=on  CountDirPort=off  CountDataType=Unsigned  CountWordLen=nextpow2(NumberOfCORDICIterations)  CountFracLen=0  CountSampTime=1
  OR : Logic  Operator=OR  IconShape=distinctive  AllPortsSameDT=off  OutDataTypeStr=boolean
  SR_latch : Subsystem
  State Control : StateControl  StateControl=Synchronous
  ValidIn to Ready Logic : Subsystem
  count_is_positive : Outport  VectorParamsAs1DForOutWhenUnconnected=off
  count : Outport  Port=2  VectorParamsAs1DForOutWhenUnconnected=off
  last : Outport  Port=3  VectorParamsAs1DForOutWhenUnconnected=off
  ready : Outport  Port=4  VectorParamsAs1DForOutWhenUnconnected=off
  wires:
  ValidIn to Ready Logic/1(readyOut) -> ready/1
  SR_latch/1(Q) -> ValidIn to Ready Logic/1(readyIn)  "ready"
  validIn/1 -> OR/2, SR_latch/2(R), ValidIn to Ready Logic/2(validIn)
  Compare To Constant/1 -> last/1, SR_latch/1(S)
  Compare To Zero/1 -> OR/1, count_is_positive/1
  OR/1 -> HDL Counter1/1
  HDL Counter1/1 -> Compare To Constant/1, count/1, Compare To Zero/1  "count"

== system MVDR_example_hdl_4x4_systolic/MVDR HDL/Compute Weight Vector/Matrix Left Divide/CORDIC/4x4 Complex CORDIC Matrix Left Divide/Q'B, R 4x4 Complex CORDIC Systolic Array/Leading Complex Row Rotation - 3/Q'B, R Row Rotations - Complex/Same Datatype ==
  Data : Inport
  Reference : Inport  Port=2
  Data Type Duplicate : DataTypeDuplicate
  DataOut : Outport  VectorParamsAs1DForOutWhenUnconnected=off
  wires:
  Data/1 -> Data Type Duplicate/1, DataOut/1
  Reference/1 -> Data Type Duplicate/2

== system MVDR_example_hdl_4x4_systolic/MVDR HDL/Compute Weight Vector/Matrix Left Divide/CORDIC/4x4 Complex CORDIC Matrix Left Divide/Q'B, R 4x4 Complex CORDIC Systolic Array/Leading Complex Row Rotation - 3/Q'B, R Row Rotations - Complex/Same Datatype1 ==
  Data : Inport
  Reference : Inport  Port=2
  Data Type Duplicate : DataTypeDuplicate
  DataOut : Outport  VectorParamsAs1DForOutWhenUnconnected=off
  wires:
  Data/1 -> Data Type Duplicate/1, DataOut/1
  Reference/1 -> Data Type Duplicate/2

== system MVDR_example_hdl_4x4_systolic/MVDR HDL/Compute Weight Vector/Matrix Left Divide/CORDIC/4x4 Complex CORDIC Matrix Left Divide/Q'B, R 4x4 Complex CORDIC Systolic Array/Leading Complex Row Rotation - 3/Q'B, R Row Rotations - Complex/Same Datatype2 ==
  Data : Inport
  Reference : Inport  Port=2
  Data Type Duplicate : DataTypeDuplicate
  DataOut : Outport  VectorParamsAs1DForOutWhenUnconnected=off
  wires:
  Data/1 -> Data Type Duplicate/1, DataOut/1
  Reference/1 -> Data Type Duplicate/2

== system MVDR_example_hdl_4x4_systolic/MVDR HDL/Compute Weight Vector/Matrix Left Divide/CORDIC/4x4 Complex CORDIC Matrix Left Divide/Q'B, R 4x4 Complex CORDIC Systolic Array/Leading Complex Row Rotation - 3/Q'B, R Row Rotations - Complex/Same Datatype3 ==
  Data : Inport
  Reference : Inport  Port=2
  Data Type Duplicate : DataTypeDuplicate
  DataOut : Outport  VectorParamsAs1DForOutWhenUnconnected=off
  wires:
  Data/1 -> Data Type Duplicate/1, DataOut/1
  Reference/1 -> Data Type Duplicate/2

== system MVDR_example_hdl_4x4_systolic/MVDR HDL/Compute Weight Vector/Matrix Left Divide/CORDIC/4x4 Complex CORDIC Matrix Left Divide/Q'B, R 4x4 Complex CORDIC Systolic Array/Leading Complex Row Rotation - 3/Rotate first element to real/Inverse CORDIC Gain1 ==
  In1 : Inport
  Inverse CORDIC Gain : Gain  Gain=1/prod(sqrt(1+2.^(-2*(0:double(NumberOfCORDICIterations)-1))))  OutDataTypeStr=Inherit: Same as input
  Out1 : Outport  VectorParamsAs1DForOutWhenUnconnected=off
  wires:
  Inverse CORDIC Gain/1 -> Out1/1
  In1/1 -> Inverse CORDIC Gain/1

== system MVDR_example_hdl_4x4_systolic/MVDR HDL/Compute Weight Vector/Matrix Left Divide/CORDIC/4x4 Complex CORDIC Matrix Left Divide/Q'B, R 4x4 Complex CORDIC Systolic Array/Leading Complex Row Rotation - 3/Rotate first element to real/Inverse CORDIC Gain2 ==
  In1 : Inport
  Inverse CORDIC Gain : Gain  Gain=1/prod(sqrt(1+2.^(-2*(0:double(NumberOfCORDICIterations)-1))))  OutDataTypeStr=Inherit: Same as input
  Out1 : Outport  VectorParamsAs1DForOutWhenUnconnected=off
  wires:
  Inverse CORDIC Gain/1 -> Out1/1
  In1/1 -> Inverse CORDIC Gain/1

== system MVDR_example_hdl_4x4_systolic/MVDR HDL/Compute Weight Vector/Matrix Left Divide/CORDIC/4x4 Complex CORDIC Matrix Left Divide/Q'B, R 4x4 Complex CORDIC Systolic Array/Leading Complex Row Rotation - 3/Rotate first element to real/Inverse CORDIC Gain3 ==
  In1 : Inport
  Inverse CORDIC Gain : Gain  Gain=1/prod(sqrt(1+2.^(-2*(0:double(NumberOfCORDICIterations)-1))))  OutDataTypeStr=Inherit: Same as input
  Out1 : Outport  VectorParamsAs1DForOutWhenUnconnected=off
  wires:
  Inverse CORDIC Gain/1 -> Out1/1
  In1/1 -> Inverse CORDIC Gain/1

== system MVDR_example_hdl_4x4_systolic/MVDR HDL/Compute Weight Vector/Matrix Left Divide/CORDIC/4x4 Complex CORDIC Matrix Left Divide/Q'B, R 4x4 Complex CORDIC Systolic Array/Leading Complex Row Rotation - 3/Rotate first element to real/Inverse CORDIC Gain4 ==
  In1 : Inport
  Inverse CORDIC Gain : Gain  Gain=1/prod(sqrt(1+2.^(-2*(0:double(NumberOfCORDICIterations)-1))))  OutDataTypeStr=Inherit: Same as input
  Out1 : Outport  VectorParamsAs1DForOutWhenUnconnected=off
  wires:
  Inverse CORDIC Gain/1 -> Out1/1
  In1/1 -> Inverse CORDIC Gain/1

== system MVDR_example_hdl_4x4_systolic/MVDR HDL/Compute Weight Vector/Matrix Left Divide/CORDIC/4x4 Complex CORDIC Matrix Left Divide/Q'B, R 4x4 Complex CORDIC Systolic Array/Leading Complex Row Rotation - 3/Rotate first element to real/Q'B, R Row Rotations - Real ==
  x : Inport
  y : Inport  Port=2
  u : Inport  Port=3
  v : Inport  Port=4
  validIn : Inport  Port=5
  CORDIC Counter : Subsystem  mask{NumberOfCORDICIterations=NumberOfCORDICIterations}
      mask prompts: NumberOfCORDICIterations "Number of CORDIC Iterations"
  Delay{1..12} (12 alike) : Delay  DelayLength=1
  Delay13 : Delay  DelayLength=1  InitialCondition=true
  MATLAB Function : MATLAB Function  TreatAsAtomicUnit=on
  Same Datatype : Subsystem  TreatAsAtomicUnit=on
  Same Datatype1 : Subsystem  TreatAsAtomicUnit=on
  Same Datatype2 : Subsystem  TreatAsAtomicUnit=on
  Same Datatype3 : Subsystem  TreatAsAtomicUnit=on
  State Control : StateControl  StateControl=Synchronous
  Switch{,1..3} (4 alike) : Switch  Criteria=u2 ~= 0
  x_out : Outport  VectorParamsAs1DForOutWhenUnconnected=off
  y_out : Outport  Port=2  VectorParamsAs1DForOutWhenUnconnected=off
  u_out : Outport  Port=3  VectorParamsAs1DForOutWhenUnconnected=off
  v_out : Outport  Port=4  VectorParamsAs1DForOutWhenUnconnected=off
  validOut : Outport  Port=5  VectorParamsAs1DForOutWhenUnconnected=off
  ready : Outport  Port=6  VectorParamsAs1DForOutWhenUnconnected=off
  wires:
  Same Datatype2/1(DataOut) -> Switch3/1
  Same Datatype3/1(DataOut) -> Switch2/1
  Same Datatype1/1(DataOut) -> Switch1/1
  Same Datatype/1(DataOut) -> Switch/1
  v/1 -> Delay8/1
  u/1 -> Delay6/1
  y/1 -> Delay5/1
  x/1 -> Delay4/1
  CORDIC Counter/1(count_is_positive) -> Delay9/1
  Switch3/1 -> MATLAB Function/4(v)
  Switch2/1 -> MATLAB Function/3(u)
  Switch1/1 -> MATLAB Function/2(y)
  Switch/1 -> MATLAB Function/1(x)
  CORDIC Counter/4(ready) -> Delay13/1
  CORDIC Counter/3(last) -> Delay12/1
  CORDIC Counter/2(count) -> Delay10/1
  validIn/1 -> CORDIC Counter/1(validIn)
  Delay3/1 -> validOut/1
  Delay7/1 -> u_out/1, Same Datatype3/1(Data)
  MATLAB Function/4(v_out) -> Delay11/1
  MATLAB Function/3(u_out) -> Delay7/1
  MATLAB Function/2(y_out) -> Delay2/1
  MATLAB Function/1(x_out) -> Delay1/1
  Delay11/1 -> v_out/1, Same Datatype2/1(Data)
  Delay2/1 -> y_out/1, Same Datatype1/1(Data)
  Delay1/1 -> x_out/1, Same Datatype/1(Data)
  Delay4/1 -> Switch/3, Same Datatype/2(Reference)
  Delay5/1 -> Switch1/3, Same Datatype1/2(Reference)
  Delay6/1 -> Switch2/3, Same Datatype3/2(Reference)
  Delay8/1 -> Switch3/3, Same Datatype2/2(Reference)
  Delay9/1 -> Switch3/2, Switch2/2, Switch1/2, Switch/2
  Delay10/1 -> MATLAB Function/5(iteration)
  Delay12/1 -> Delay3/1
  Delay13/1 -> ready/1

== system MVDR_example_hdl_4x4_systolic/MVDR HDL/Compute Weight Vector/Matrix Left Divide/CORDIC/4x4 Complex CORDIC Matrix Left Divide/Q'B, R 4x4 Complex CORDIC Systolic Array/Leading Complex Row Rotation - 3/Rotate first element to real/ValidIn to Ready Logic with Delay ==
  readyIn : Inport
  validIn * z^-1 : Inport  Port=2
  validIn : Inport  Port=3
  AND : Logic  IconShape=distinctive  AllPortsSameDT=off  OutDataTypeStr=boolean
  AND1 : Logic  IconShape=distinctive  AllPortsSameDT=off  OutDataTypeStr=boolean
  NOT : Logic  Operator=NOT  IconShape=distinctive  AllPortsSameDT=off  OutDataTypeStr=boolean
  NOT1 : Logic  Operator=NOT  IconShape=distinctive  AllPortsSameDT=off  OutDataTypeStr=boolean
  readyOut : Outport  VectorParamsAs1DForOutWhenUnconnected=off
  wires:
  validIn * z^-1/1 -> NOT/1
  validIn/1 -> NOT1/1
  readyIn/1 -> AND/1
  AND1/1 -> readyOut/1
  NOT1/1 -> AND1/2
  NOT/1 -> AND/2
  AND/1 -> AND1/1

== system MVDR_example_hdl_4x4_systolic/MVDR HDL/Compute Weight Vector/Matrix Left Divide/CORDIC/4x4 Complex CORDIC Matrix Left Divide/Q'B, R 4x4 Complex CORDIC Systolic Array/Leading Complex Row Rotation - 3/Rotate first element to real - 1/Inverse CORDIC Gain1 ==
  In1 : Inport
  Inverse CORDIC Gain : Gain  Gain=1/prod(sqrt(1+2.^(-2*(0:double(NumberOfCORDICIterations)-1))))  OutDataTypeStr=Inherit: Same as input
  Out1 : Outport  VectorParamsAs1DForOutWhenUnconnected=off
  wires:
  Inverse CORDIC Gain/1 -> Out1/1
  In1/1 -> Inverse CORDIC Gain/1

== system MVDR_example_hdl_4x4_systolic/MVDR HDL/Compute Weight Vector/Matrix Left Divide/CORDIC/4x4 Complex CORDIC Matrix Left Divide/Q'B, R 4x4 Complex CORDIC Systolic Array/Leading Complex Row Rotation - 3/Rotate first element to real - 1/Inverse CORDIC Gain2 ==
  In1 : Inport
  Inverse CORDIC Gain : Gain  Gain=1/prod(sqrt(1+2.^(-2*(0:double(NumberOfCORDICIterations)-1))))  OutDataTypeStr=Inherit: Same as input
  Out1 : Outport  VectorParamsAs1DForOutWhenUnconnected=off
  wires:
  Inverse CORDIC Gain/1 -> Out1/1
  In1/1 -> Inverse CORDIC Gain/1

== system MVDR_example_hdl_4x4_systolic/MVDR HDL/Compute Weight Vector/Matrix Left Divide/CORDIC/4x4 Complex CORDIC Matrix Left Divide/Q'B, R 4x4 Complex CORDIC Systolic Array/Leading Complex Row Rotation - 3/Rotate first element to real - 1/Inverse CORDIC Gain3 ==
  In1 : Inport
  Inverse CORDIC Gain : Gain  Gain=1/prod(sqrt(1+2.^(-2*(0:double(NumberOfCORDICIterations)-1))))  OutDataTypeStr=Inherit: Same as input
  Out1 : Outport  VectorParamsAs1DForOutWhenUnconnected=off
  wires:
  Inverse CORDIC Gain/1 -> Out1/1
  In1/1 -> Inverse CORDIC Gain/1

== system MVDR_example_hdl_4x4_systolic/MVDR HDL/Compute Weight Vector/Matrix Left Divide/CORDIC/4x4 Complex CORDIC Matrix Left Divide/Q'B, R 4x4 Complex CORDIC Systolic Array/Leading Complex Row Rotation - 3/Rotate first element to real - 1/Inverse CORDIC Gain4 ==
  In1 : Inport
  Inverse CORDIC Gain : Gain  Gain=1/prod(sqrt(1+2.^(-2*(0:double(NumberOfCORDICIterations)-1))))  OutDataTypeStr=Inherit: Same as input
  Out1 : Outport  VectorParamsAs1DForOutWhenUnconnected=off
  wires:
  Inverse CORDIC Gain/1 -> Out1/1
  In1/1 -> Inverse CORDIC Gain/1

== system MVDR_example_hdl_4x4_systolic/MVDR HDL/Compute Weight Vector/Matrix Left Divide/CORDIC/4x4 Complex CORDIC Matrix Left Divide/Q'B, R 4x4 Complex CORDIC Systolic Array/Leading Complex Row Rotation - 3/Rotate first element to real - 1/Q'B, R Row Rotations - Real ==
  x : Inport
  y : Inport  Port=2
  u : Inport  Port=3
  v : Inport  Port=4
  validIn : Inport  Port=5
  CORDIC Counter : Subsystem  mask{NumberOfCORDICIterations=NumberOfCORDICIterations}
      mask prompts: NumberOfCORDICIterations "Number of CORDIC Iterations"
  Delay{1..12} (12 alike) : Delay  DelayLength=1
  Delay13 : Delay  DelayLength=1  InitialCondition=true
  MATLAB Function : MATLAB Function  TreatAsAtomicUnit=on
  Same Datatype : Subsystem  TreatAsAtomicUnit=on
  Same Datatype1 : Subsystem  TreatAsAtomicUnit=on
  Same Datatype2 : Subsystem  TreatAsAtomicUnit=on
  Same Datatype3 : Subsystem  TreatAsAtomicUnit=on
  State Control : StateControl  StateControl=Synchronous
  Switch{,1..3} (4 alike) : Switch  Criteria=u2 ~= 0
  x_out : Outport  VectorParamsAs1DForOutWhenUnconnected=off
  y_out : Outport  Port=2  VectorParamsAs1DForOutWhenUnconnected=off
  u_out : Outport  Port=3  VectorParamsAs1DForOutWhenUnconnected=off
  v_out : Outport  Port=4  VectorParamsAs1DForOutWhenUnconnected=off
  validOut : Outport  Port=5  VectorParamsAs1DForOutWhenUnconnected=off
  ready : Outport  Port=6  VectorParamsAs1DForOutWhenUnconnected=off
  wires:
  Delay13/1 -> ready/1
  Delay12/1 -> Delay3/1
  Delay10/1 -> MATLAB Function/5(iteration)
  Delay9/1 -> Switch/2, Switch1/2, Switch2/2, Switch3/2
  Delay8/1 -> Same Datatype2/2(Reference), Switch3/3
  Delay6/1 -> Same Datatype3/2(Reference), Switch2/3
  Delay5/1 -> Same Datatype1/2(Reference), Switch1/3
  Delay4/1 -> Same Datatype/2(Reference), Switch/3
  Delay1/1 -> Same Datatype/1(Data), x_out/1
  Delay2/1 -> Same Datatype1/1(Data), y_out/1
  Delay11/1 -> Same Datatype2/1(Data), v_out/1
  MATLAB Function/1(x_out) -> Delay1/1
  MATLAB Function/2(y_out) -> Delay2/1
  MATLAB Function/3(u_out) -> Delay7/1
  MATLAB Function/4(v_out) -> Delay11/1
  Delay7/1 -> Same Datatype3/1(Data), u_out/1
  Delay3/1 -> validOut/1
  validIn/1 -> CORDIC Counter/1(validIn)
  CORDIC Counter/2(count) -> Delay10/1
  CORDIC Counter/3(last) -> Delay12/1
  CORDIC Counter/4(ready) -> Delay13/1
  Switch/1 -> MATLAB Function/1(x)
  Switch1/1 -> MATLAB Function/2(y)
  Switch2/1 -> MATLAB Function/3(u)
  Switch3/1 -> MATLAB Function/4(v)
  CORDIC Counter/1(count_is_positive) -> Delay9/1
  x/1 -> Delay4/1
  y/1 -> Delay5/1
  u/1 -> Delay6/1
  v/1 -> Delay8/1
  Same Datatype/1(DataOut) -> Switch/1
  Same Datatype1/1(DataOut) -> Switch1/1
  Same Datatype3/1(DataOut) -> Switch2/1
  Same Datatype2/1(DataOut) -> Switch3/1

== system MVDR_example_hdl_4x4_systolic/MVDR HDL/Compute Weight Vector/Matrix Left Divide/CORDIC/4x4 Complex CORDIC Matrix Left Divide/Q'B, R 4x4 Complex CORDIC Systolic Array/Leading Complex Row Rotation - 3/Rotate first element to real - 1/ValidIn to Ready Logic with Delay ==
  readyIn : Inport
  validIn * z^-1 : Inport  Port=2
  validIn : Inport  Port=3
  AND : Logic  IconShape=distinctive  AllPortsSameDT=off  OutDataTypeStr=boolean
  AND1 : Logic  IconShape=distinctive  AllPortsSameDT=off  OutDataTypeStr=boolean
  NOT : Logic  Operator=NOT  IconShape=distinctive  AllPortsSameDT=off  OutDataTypeStr=boolean
  NOT1 : Logic  Operator=NOT  IconShape=distinctive  AllPortsSameDT=off  OutDataTypeStr=boolean
  readyOut : Outport  VectorParamsAs1DForOutWhenUnconnected=off
  wires:
  validIn * z^-1/1 -> NOT/1
  validIn/1 -> NOT1/1
  readyIn/1 -> AND/1
  AND1/1 -> readyOut/1
  NOT1/1 -> AND1/2
  NOT/1 -> AND/2
  AND/1 -> AND1/1

== system MVDR_example_hdl_4x4_systolic/MVDR HDL/Compute Weight Vector/Matrix Left Divide/CORDIC/4x4 Complex CORDIC Matrix Left Divide/Q'B, R 4x4 Complex CORDIC Systolic Array/Leading Complex Row Rotation - 4/Q'B, R Row Rotations - Complex/CORDIC Counter ==
  validIn : Inport
  Compare To Constant : simulink/Logic and Bit Operations/Compare To Constant  relop===  const=NumberOfCORDICIterations-1  OutDataTypeStr=boolean
  Compare To Zero : simulink/Logic and Bit Operations/Compare To Zero  relop=>  OutDataTypeStr=boolean
  HDL Counter1 : hdlsllib/Sources/HDL Counter  CountType=Count limited  CountInit=0  CountStep=1  CountMax=NumberOfCORDICIterations-1  CountFromType=Initial value  CountFrom=0  CountResetPort=off  CountLoadPort=off  CountEnbPort=on  CountDirPort=off  CountDataType=Unsigned  CountWordLen=nextpow2(NumberOfCORDICIterations)  CountFracLen=0  CountSampTime=1
  OR : Logic  Operator=OR  IconShape=distinctive  AllPortsSameDT=off  OutDataTypeStr=boolean
  SR_latch : Subsystem
  State Control : StateControl  StateControl=Synchronous
  ValidIn to Ready Logic : Subsystem
  count_is_positive : Outport  VectorParamsAs1DForOutWhenUnconnected=off
  count : Outport  Port=2  VectorParamsAs1DForOutWhenUnconnected=off
  last : Outport  Port=3  VectorParamsAs1DForOutWhenUnconnected=off
  ready : Outport  Port=4  VectorParamsAs1DForOutWhenUnconnected=off
  wires:
  ValidIn to Ready Logic/1(readyOut) -> ready/1
  SR_latch/1(Q) -> ValidIn to Ready Logic/1(readyIn)  "ready"
  validIn/1 -> OR/2, SR_latch/2(R), ValidIn to Ready Logic/2(validIn)
  Compare To Constant/1 -> last/1, SR_latch/1(S)
  Compare To Zero/1 -> OR/1, count_is_positive/1
  OR/1 -> HDL Counter1/1
  HDL Counter1/1 -> Compare To Constant/1, count/1, Compare To Zero/1  "count"

== system MVDR_example_hdl_4x4_systolic/MVDR HDL/Compute Weight Vector/Matrix Left Divide/CORDIC/4x4 Complex CORDIC Matrix Left Divide/Q'B, R 4x4 Complex CORDIC Systolic Array/Leading Complex Row Rotation - 4/Q'B, R Row Rotations - Complex/Same Datatype ==
  Data : Inport
  Reference : Inport  Port=2
  Data Type Duplicate : DataTypeDuplicate
  DataOut : Outport  VectorParamsAs1DForOutWhenUnconnected=off
  wires:
  Data/1 -> Data Type Duplicate/1, DataOut/1
  Reference/1 -> Data Type Duplicate/2

== system MVDR_example_hdl_4x4_systolic/MVDR HDL/Compute Weight Vector/Matrix Left Divide/CORDIC/4x4 Complex CORDIC Matrix Left Divide/Q'B, R 4x4 Complex CORDIC Systolic Array/Leading Complex Row Rotation - 4/Q'B, R Row Rotations - Complex/Same Datatype1 ==
  Data : Inport
  Reference : Inport  Port=2
  Data Type Duplicate : DataTypeDuplicate
  DataOut : Outport  VectorParamsAs1DForOutWhenUnconnected=off
  wires:
  Data/1 -> Data Type Duplicate/1, DataOut/1
  Reference/1 -> Data Type Duplicate/2

== system MVDR_example_hdl_4x4_systolic/MVDR HDL/Compute Weight Vector/Matrix Left Divide/CORDIC/4x4 Complex CORDIC Matrix Left Divide/Q'B, R 4x4 Complex CORDIC Systolic Array/Leading Complex Row Rotation - 4/Q'B, R Row Rotations - Complex/Same Datatype2 ==
  Data : Inport
  Reference : Inport  Port=2
  Data Type Duplicate : DataTypeDuplicate
  DataOut : Outport  VectorParamsAs1DForOutWhenUnconnected=off
  wires:
  Data/1 -> Data Type Duplicate/1, DataOut/1
  Reference/1 -> Data Type Duplicate/2

== system MVDR_example_hdl_4x4_systolic/MVDR HDL/Compute Weight Vector/Matrix Left Divide/CORDIC/4x4 Complex CORDIC Matrix Left Divide/Q'B, R 4x4 Complex CORDIC Systolic Array/Leading Complex Row Rotation - 4/Q'B, R Row Rotations - Complex/Same Datatype3 ==
  Data : Inport
  Reference : Inport  Port=2
  Data Type Duplicate : DataTypeDuplicate
  DataOut : Outport  VectorParamsAs1DForOutWhenUnconnected=off
  wires:
  Data/1 -> Data Type Duplicate/1, DataOut/1
  Reference/1 -> Data Type Duplicate/2

== system MVDR_example_hdl_4x4_systolic/MVDR HDL/Compute Weight Vector/Matrix Left Divide/CORDIC/4x4 Complex CORDIC Matrix Left Divide/Q'B, R 4x4 Complex CORDIC Systolic Array/Leading Complex Row Rotation - 4/Rotate first element to real/Inverse CORDIC Gain1 ==
  In1 : Inport
  Inverse CORDIC Gain : Gain  Gain=1/prod(sqrt(1+2.^(-2*(0:double(NumberOfCORDICIterations)-1))))  OutDataTypeStr=Inherit: Same as input
  Out1 : Outport  VectorParamsAs1DForOutWhenUnconnected=off
  wires:
  Inverse CORDIC Gain/1 -> Out1/1
  In1/1 -> Inverse CORDIC Gain/1

== system MVDR_example_hdl_4x4_systolic/MVDR HDL/Compute Weight Vector/Matrix Left Divide/CORDIC/4x4 Complex CORDIC Matrix Left Divide/Q'B, R 4x4 Complex CORDIC Systolic Array/Leading Complex Row Rotation - 4/Rotate first element to real/Inverse CORDIC Gain2 ==
  In1 : Inport
  Inverse CORDIC Gain : Gain  Gain=1/prod(sqrt(1+2.^(-2*(0:double(NumberOfCORDICIterations)-1))))  OutDataTypeStr=Inherit: Same as input
  Out1 : Outport  VectorParamsAs1DForOutWhenUnconnected=off
  wires:
  Inverse CORDIC Gain/1 -> Out1/1
  In1/1 -> Inverse CORDIC Gain/1

== system MVDR_example_hdl_4x4_systolic/MVDR HDL/Compute Weight Vector/Matrix Left Divide/CORDIC/4x4 Complex CORDIC Matrix Left Divide/Q'B, R 4x4 Complex CORDIC Systolic Array/Leading Complex Row Rotation - 4/Rotate first element to real/Inverse CORDIC Gain3 ==
  In1 : Inport
  Inverse CORDIC Gain : Gain  Gain=1/prod(sqrt(1+2.^(-2*(0:double(NumberOfCORDICIterations)-1))))  OutDataTypeStr=Inherit: Same as input
  Out1 : Outport  VectorParamsAs1DForOutWhenUnconnected=off
  wires:
  Inverse CORDIC Gain/1 -> Out1/1
  In1/1 -> Inverse CORDIC Gain/1

== system MVDR_example_hdl_4x4_systolic/MVDR HDL/Compute Weight Vector/Matrix Left Divide/CORDIC/4x4 Complex CORDIC Matrix Left Divide/Q'B, R 4x4 Complex CORDIC Systolic Array/Leading Complex Row Rotation - 4/Rotate first element to real/Inverse CORDIC Gain4 ==
  In1 : Inport
  Inverse CORDIC Gain : Gain  Gain=1/prod(sqrt(1+2.^(-2*(0:double(NumberOfCORDICIterations)-1))))  OutDataTypeStr=Inherit: Same as input
  Out1 : Outport  VectorParamsAs1DForOutWhenUnconnected=off
  wires:
  Inverse CORDIC Gain/1 -> Out1/1
  In1/1 -> Inverse CORDIC Gain/1
